simulink model "parte2"  (R2015a)
settings: Solver=ode3  StartTime=0.0  StopTime=30  RelTol=1e-3
values from neighbouring files (symbols this model uses):
  Nbar = inv(C*inv(eye(size(A)) - A + B*K)*B)    [parte2.m]
undefined symbols (not defined in the file or in its folder): A, B, C, D, K, Ke, Kp, M, MIO, National_Instruments, PCI, sampling_time
libraries: sldrtlib x3
settings Model: SimulationMode=external  ExtModeTrigDuration=300000  Creator=Alunos  LastModifiedBy=Alunos
settings HardwareCC: ProdIntDivRoundTo=Zero  ProdEndianess=LittleEndian  ProdHWDeviceType=Intel->x86/Pentium  TargetIntDivRoundTo=Zero  TargetEndianess=LittleEndian  TargetHWDeviceType=Intel->x86/Pentium
settings RTWCC: SystemTargetFile=rtwin.tlc  TemplateMakefile=rtwin.tmf  Description=Simulink Desktop Real-Time  RTWCompilerOptimization=on
settings CodeAppCC: MaxIdLength=95
settings RTWinTargetCC: TargetPreCompLibLocation=C:\Program Files\MATLAB\R2015a\toolbox\sldrt\lib\win32

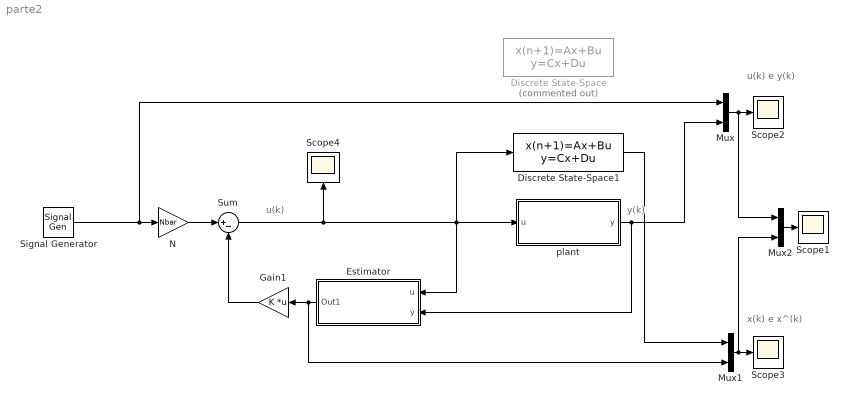
== system parte2 ==
  note: y(k)
  note: x(k) e x^(k)
  note: u(k) e y(k)
  note: u(k)
  Discrete State-Space : DiscreteStateSpace  Commented=on  A=A  B=B  C=C  D=D  SampleTime=sampling_time
  Discrete State-Space1 : DiscreteStateSpace  A=A  B=B  C=ones(size(C))  D=0  SampleTime=sampling_time
  Estimator : Subsystem
  Gain1 : Gain  Gain=K  Multiplication=Matrix(K*u)
  Mux : Mux  Inputs=2
  Mux1 : Mux  Inputs=2
  Mux2 : Mux  Inputs=2
  N : Gain  Gain=Nbar
  Scope{1..4} (4 alike) : Scope
      Scope1 settings: YMin=-525  YMax=0
      Scope2 settings: YMin=-47  YMax=-30
      Scope3 settings: YMin=-525  YMax=0  SaveName=ScopeData2
      Scope4 settings: YMin=-4.25  YMax=0.25  SaveName=ScopeData3
  Signal Generator : SignalGenerator  Amplitude=45  Frequency=0.25
  Sum : Sum  Inputs=|+-
  plant : Subsystem
  wires:
  Signal Generator/1 -> Mux/1, N/1
  Estimator/1(Out1) -> Mux1/2, Gain1/1
  N/1 -> Sum/1
  Gain1/1 -> Sum/2
  Sum/1 -> Discrete State-Space1/1, plant/1("u "), Estimator/1("u "), Scope4/1
  Discrete State-Space1/1 -> Mux1/1
  Mux/1 -> Mux2/1, Scope2/1
  Mux1/1 -> Mux2/2, Scope3/1
  Mux2/1 -> Scope1/1
  plant/1("y ") -> Estimator/2(y), Mux/2

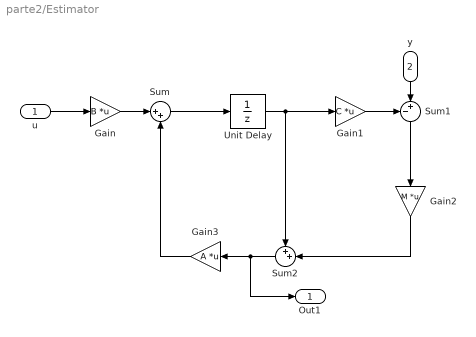
== system parte2/Estimator ==
  "u " : Inport
  y : Inport  Port=2
  Gain : Gain  Gain=B  Multiplication=Matrix(K*u)
  Gain1 : Gain  Gain=C  Multiplication=Matrix(K*u)
  Gain2 : Gain  Gain=M  Multiplication=Matrix(K*u)
  Gain3 : Gain  Gain=A  Multiplication=Matrix(K*u)
  Sum : Sum  Inputs=|++
  Sum1 : Sum  Inputs=-+|
  Sum2 : Sum  Inputs=++|
  Unit Delay : UnitDelay  SampleTime=sampling_time
  Out1 : Outport
  wires:
  y/1 -> Sum1/2
  Gain1/1 -> Sum1/1
  Sum1/1 -> Gain2/1
  Gain3/1 -> Sum/2
  Gain2/1 -> Sum2/2
  Sum2/1 -> Out1/1, Gain3/1
  Unit Delay/1 -> Sum2/1, Gain1/1
  Sum/1 -> Unit Delay/1
  Gain/1 -> Sum/1
  "u "/1 -> Gain/1

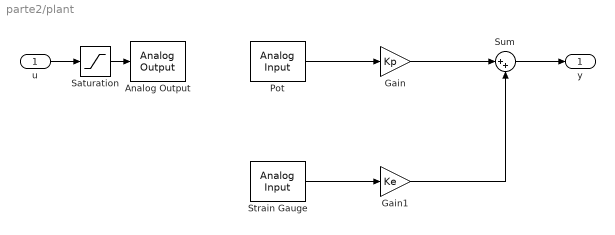
== system parte2/plant ==
  "u " : Inport
  Analog Output : sldrtlib/Analog Output  SampleTime=sampling_time  MaxMissedTicks=10  ShowMissedTicks=off  YieldWhenWaiting=off  DrvName=National_Instruments/PCI-MIO-16E-4  DrvAddress=4294967295  DrvOptions=[0 0 0 0 0 0]  Channels=1  RangeMode=1  VoltRange=1  InitialValue=0  FinalValue=0
      settings: AttributesFormatString=National Instruments\nPCI-MIO-16E-4 [auto]
  Gain : Gain  Gain=Kp
  Gain1 : Gain  Gain=Ke
  Pot : sldrtlib/Analog Input  SampleTime=sampling_time  MaxMissedTicks=10  ShowMissedTicks=off  YieldWhenWaiting=off  DrvName=National_Instruments/PCI-MIO-16E-4  DrvAddress=4294967295  DrvOptions=[0 0 0 0 0 0]  Channels=1  RangeMode=1  VoltRange=1  DataType=1
      settings: AttributesFormatString=National Instruments\nPCI-MIO-16E-4 [auto]
  Saturation : Saturate  UpperLimit=5  LowerLimit=-5
  Strain Gauge : sldrtlib/Analog Input  SampleTime=sampling_time  MaxMissedTicks=10  ShowMissedTicks=off  YieldWhenWaiting=off  DrvName=National_Instruments/PCI-MIO-16E-4  DrvAddress=4294967295  DrvOptions=[0 0 0 0 0 0]  Channels=2  RangeMode=1  VoltRange=1  DataType=1
      settings: AttributesFormatString=National Instruments\nPCI-MIO-16E-4 [auto]
  Sum : Sum  Inputs=|++
  "y " : Outport
  wires:
  Gain1/1 -> Sum/2
  Pot/1 -> Gain/1
  Strain Gauge/1 -> Gain1/1
  Gain/1 -> Sum/1
  Sum/1 -> "y "/1
  "u "/1 -> Saturation/1
  Saturation/1 -> Analog Output/1
